simulink model "PV_Series_Parallel_Array"  (R2020a)
settings: Solver=VariableStepAuto  StartTime=0.0  StopTime=5  RelTol=1e-3
values from neighbouring files (symbols this model uses):
  Eg = 1.1    [data.m]
  Isc = 8.21    [data.m]
  k = 1.38*((10)^-23)    (= 1.38e-23)    [data.m]
  ki = 0.0032    [data.m]
  n = 1.3    [data.m]
  Ns = 54    [data.m]
  q = 1.6*((10)^-19)    (= 1.6e-19)    [data.m]
  Rs = 0.221    [data.m]
  Rsh = 415.405    [data.m]
  Tn = 298    [data.m]
  Voc = 32.9    [data.m]
libraries: powerlib x25
settings Model: Creator=Khojasteh Mirza  LastModifiedBy=Khojasteh Mirza

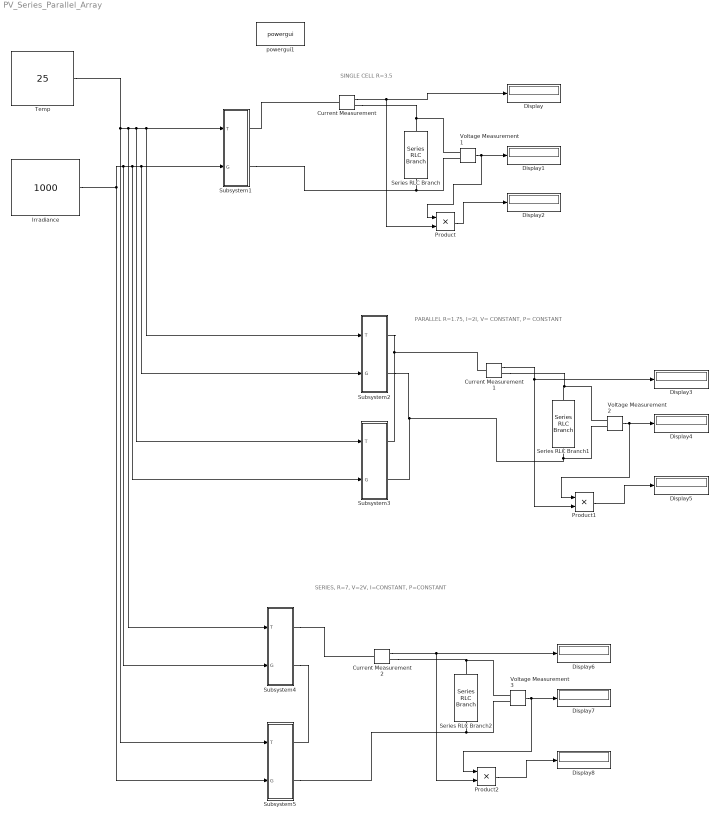
== system PV_Series_Parallel_Array ==
  note: SERIES, R=7, V=2V, I=CONSTANT, P=CONSTANT
  note: PARALLEL R=1.75, I=2I, V= CONSTANT, P= CONSTANT
  note: SINGLE CELL R=3.5
  Current Measurement : powerlib/Measurements/Current Measurement  PhasorSimulation=off  OutputType=Complex  PSBequivalent=0
  Current Measurement1 : powerlib/Measurements/Current Measurement  PhasorSimulation=off  OutputType=Complex  PSBequivalent=0
  Current Measurement2 : powerlib/Measurements/Current Measurement  PhasorSimulation=off  OutputType=Complex  PSBequivalent=0
  Display{,1..8} (9 alike) : Display
  Irradiance : Constant  Value=1000
  Product : Product
  Product1 : Product
  Product2 : Product
  Series RLC Branch : powerlib/Elements/Series RLC Branch  LConnTagsString=__new0  RConnTagsString=__new0  BranchType=R  Resistance=3.5  Inductance=1e-3  SetiL0=off  InitialCurrent=0  Capacitance=1e-6  Setx0=off  InitialVoltage=0  Measurements=None
  Series RLC Branch1 : powerlib/Elements/Series RLC Branch  LConnTagsString=__new0  RConnTagsString=__new0  BranchType=R  Resistance=1.75  Inductance=1e-3  SetiL0=off  InitialCurrent=0  Capacitance=1e-6  Setx0=off  InitialVoltage=0  Measurements=None
  Series RLC Branch2 : powerlib/Elements/Series RLC Branch  LConnTagsString=__new0  RConnTagsString=__new0  BranchType=R  Resistance=7  Inductance=1e-3  SetiL0=off  InitialCurrent=0  Capacitance=1e-6  Setx0=off  InitialVoltage=0  Measurements=None
  Subsystem1 : Subsystem
  Subsystem2 : Subsystem
  Subsystem3 : Subsystem
  Subsystem4 : Subsystem
  Subsystem5 : Subsystem
  Temp : Constant  Value=25
  Voltage Measurement1 : powerlib/Measurements/Voltage Measurement  PhasorSimulation=off  OutputType=Complex  PSBequivalent=0
  Voltage Measurement2 : powerlib/Measurements/Voltage Measurement  PhasorSimulation=off  OutputType=Complex  PSBequivalent=0
  Voltage Measurement3 : powerlib/Measurements/Voltage Measurement  PhasorSimulation=off  OutputType=Complex  PSBequivalent=0
  powergui1 : powerlib/powergui  Priority=1  SimulationMode=Continuous  SampleTime=50e-6  frequency=60  Iterations=50  frequencyindice=0  Pbase=100e6  ErrMax=1e-4  UnitsV=kV  UnitsW=MW  buscounter=0  FunctionMessages=off  echomessages=off  EnableUseOfTLC=off  CurrentSourceSwitches=off  DisableSnubberDevices=off  DisableRonSwitches=off  DisableVfSwitches=off  DisplayEquations=off  AutomaticDiscreteSolvers=off  SolverType=Tustin/Backward Euler (TBE)  Interpol=off  ExternalGateDelay=off  methode=off  Ts=100  x0status=blocks  SPID=on  SwTol=0  HookPort=off  NonlinearTolerance=1e-4  nMaxIteration=100  ContinueOnMaxIteration=off  RestoreLinks=warning  ResistiveCurrentMeasurement=off  Frange=[0:2:500]  Ylog=off  Xlog=on  ShowGrid=off  save=off  variable=ZData  structure=0  ZoomFFT=off  StartTime=0.0  cycles=1  DisplayStyle=1  fundamental=60  FreqAxis=off  MaxFrequency=1000  frequencyindicesteady=1  RmsSteady=1  display=off
  wires:
  Voltage Measurement1/1 -> Product/1, Display1/1
  Current Measurement/1 -> Product/2, Display/1
  Product/1 -> Display2/1
  Irradiance/1 -> Subsystem3/2(G), Subsystem2/2(G), Subsystem1/2(G), Subsystem4/2(G), Subsystem5/2(G)
  Temp/1 -> Subsystem5/1(T), Subsystem4/1(T), Subsystem3/1(T), Subsystem2/1(T), Subsystem1/1(T)
  Product1/1 -> Display5/1
  Current Measurement1/1 -> Display3/1, Product1/2
  Voltage Measurement2/1 -> Display4/1, Product1/1
  Voltage Measurement3/1 -> Product2/1, Display7/1
  Current Measurement2/1 -> Product2/2, Display6/1
  Product2/1 -> Display8/1
  connections:
  Subsystem1/RConn2 -- Voltage Measurement1/LConn2 -- Series RLC Branch/RConn1
  Voltage Measurement1/LConn1 -- Current Measurement/RConn1 -- Series RLC Branch/LConn1
  Current Measurement/LConn1 -- Subsystem1/RConn1
  Subsystem2/RConn1 -- Subsystem3/RConn1 -- Current Measurement1/LConn1
  Voltage Measurement2/LConn2 -- Subsystem3/RConn2 -- Subsystem2/RConn2 -- Series RLC Branch1/RConn1
  Current Measurement1/RConn1 -- Voltage Measurement2/LConn1 -- Series RLC Branch1/LConn1
  Voltage Measurement3/LConn1 -- Current Measurement2/RConn1 -- Series RLC Branch2/LConn1
  Voltage Measurement3/LConn2 -- Subsystem5/RConn2 -- Series RLC Branch2/RConn1
  Subsystem4/RConn1 -- Current Measurement2/LConn1
  Subsystem4/RConn2 -- Subsystem5/RConn1

== system PV_Series_Parallel_Array/Subsystem1 ==
  T : Inport
  G : Inport  Port=2
  Controlled Current Source : powerlib/Electrical Sources/Controlled Current Source  Initialize=on  Source_Type=AC  Amplitude=0  Phase=0  Frequency=0  Measurements=None
  Diode : powerlib/Power Electronics/Diode  Ron=0.001  Lon=0  Vf=0.8  IC=0  UseSnubber=0  Rs=500  Cs=250e-9  Measurements=off
  PV Module : Subsystem
  Voltage Measurement : powerlib/Measurements/Voltage Measurement  PhasorSimulation=off  OutputType=Complex  PSBequivalent=0
  + : PMIOPort  Side=Right
  - : PMIOPort  Port=2  Side=Right
  wires:
  G/1 -> PV Module/2(G)
  Voltage Measurement/1 -> PV Module/3(Varray)
  T/1 -> PV Module/1(T)
  PV Module/1(I) -> Controlled Current Source/1
  connections:
  Voltage Measurement/LConn2 -- Diode/LConn1 -- Controlled Current Source/LConn1 -- -/RConn1
  Voltage Measurement/LConn1 -- Diode/RConn1 -- Controlled Current Source/RConn1 -- +/RConn1

== system PV_Series_Parallel_Array/Subsystem2 ==
  T : Inport
  G : Inport  Port=2
  Controlled Current Source : powerlib/Electrical Sources/Controlled Current Source  Initialize=on  Source_Type=AC  Amplitude=0  Phase=0  Frequency=0  Measurements=None
  Diode : powerlib/Power Electronics/Diode  Ron=0.001  Lon=0  Vf=0.8  IC=0  UseSnubber=0  Rs=500  Cs=250e-9  Measurements=off
  PV Module : Subsystem
  Voltage Measurement : powerlib/Measurements/Voltage Measurement  PhasorSimulation=off  OutputType=Complex  PSBequivalent=0
  + : PMIOPort  Side=Right
  - : PMIOPort  Port=2  Side=Right
  wires:
  PV Module/1(I) -> Controlled Current Source/1
  T/1 -> PV Module/1(T)
  Voltage Measurement/1 -> PV Module/3(Varray)
  G/1 -> PV Module/2(G)
  connections:
  Diode/RConn1 -- +/RConn1 -- Voltage Measurement/LConn1 -- Controlled Current Source/RConn1
  Diode/LConn1 -- Controlled Current Source/LConn1 -- -/RConn1 -- Voltage Measurement/LConn2

== system PV_Series_Parallel_Array/Subsystem3 ==
  T : Inport
  G : Inport  Port=2
  Controlled Current Source : powerlib/Electrical Sources/Controlled Current Source  Initialize=on  Source_Type=AC  Amplitude=0  Phase=0  Frequency=0  Measurements=None
  Diode : powerlib/Power Electronics/Diode  Ron=0.001  Lon=0  Vf=0.8  IC=0  UseSnubber=0  Rs=500  Cs=250e-9  Measurements=off
  PV Module : Subsystem
  Voltage Measurement : powerlib/Measurements/Voltage Measurement  PhasorSimulation=off  OutputType=Complex  PSBequivalent=0
  + : PMIOPort  Side=Right
  - : PMIOPort  Port=2  Side=Right
  wires:
  G/1 -> PV Module/2(G)
  Voltage Measurement/1 -> PV Module/3(Varray)
  T/1 -> PV Module/1(T)
  PV Module/1(I) -> Controlled Current Source/1
  connections:
  Voltage Measurement/LConn2 -- -/RConn1 -- Controlled Current Source/LConn1 -- Diode/LConn1
  Controlled Current Source/RConn1 -- Voltage Measurement/LConn1 -- +/RConn1 -- Diode/RConn1

== system PV_Series_Parallel_Array/Subsystem4 ==
  T : Inport
  G : Inport  Port=2
  Controlled Current Source : powerlib/Electrical Sources/Controlled Current Source  Initialize=on  Source_Type=AC  Amplitude=0  Phase=0  Frequency=0  Measurements=None
  Diode : powerlib/Power Electronics/Diode  Ron=0.001  Lon=0  Vf=0.8  IC=0  UseSnubber=0  Rs=500  Cs=250e-9  Measurements=off
  PV Module : Subsystem
  Voltage Measurement : powerlib/Measurements/Voltage Measurement  PhasorSimulation=off  OutputType=Complex  PSBequivalent=0
  + : PMIOPort  Side=Right
  - : PMIOPort  Port=2  Side=Right
  wires:
  G/1 -> PV Module/2(G)
  Voltage Measurement/1 -> PV Module/3(Varray)
  T/1 -> PV Module/1(T)
  PV Module/1(I) -> Controlled Current Source/1
  connections:
  Voltage Measurement/LConn2 -- -/RConn1 -- Controlled Current Source/LConn1 -- Diode/LConn1
  Controlled Current Source/RConn1 -- Voltage Measurement/LConn1 -- +/RConn1 -- Diode/RConn1

== system PV_Series_Parallel_Array/Subsystem5 ==
  T : Inport
  G : Inport  Port=2
  Controlled Current Source : powerlib/Electrical Sources/Controlled Current Source  Initialize=on  Source_Type=AC  Amplitude=0  Phase=0  Frequency=0  Measurements=None
  Diode : powerlib/Power Electronics/Diode  Ron=0.001  Lon=0  Vf=0.8  IC=0  UseSnubber=0  Rs=500  Cs=250e-9  Measurements=off
  PV Module : Subsystem
  Voltage Measurement : powerlib/Measurements/Voltage Measurement  PhasorSimulation=off  OutputType=Complex  PSBequivalent=0
  + : PMIOPort  Side=Right
  - : PMIOPort  Port=2  Side=Right
  wires:
  PV Module/1(I) -> Controlled Current Source/1
  T/1 -> PV Module/1(T)
  Voltage Measurement/1 -> PV Module/3(Varray)
  G/1 -> PV Module/2(G)
  connections:
  Diode/RConn1 -- +/RConn1 -- Voltage Measurement/LConn1 -- Controlled Current Source/RConn1
  Diode/LConn1 -- Controlled Current Source/LConn1 -- -/RConn1 -- Voltage Measurement/LConn2

== system PV_Series_Parallel_Array/Subsystem1/PV Module ==
  T : Inport
  G : Inport  Port=2
  Varray : Inport  Port=3
  Add : Sum
  Constant : Constant  Value=273
  PV Current : Subsystem
  Photo current : Subsystem
  Reverse Saturation Current : Subsystem
  Saturation Current : Subsystem
  Shunt Current : Subsystem
  I : Outport
  wires:
  Shunt Current/1(Ish) -> PV Current/4(Ish)
  Varray/1 -> Shunt Current/2(V), PV Current/1(V)
  Reverse Saturation Current/1(Irs) -> Saturation Current/2(Irs)
  Saturation Current/1(I_0) -> PV Current/3(I0)
  Constant/1 -> Add/2
  G/1 -> Photo current/2(G)
  T/1 -> Add/1
  PV Current/1(I) -> I/1, Shunt Current/1(I)
  Photo current/1(Iph) -> PV Current/5(Iph)
  Add/1 -> Saturation Current/1(T), Reverse Saturation Current/1(T), Photo current/1(T), PV Current/2(T)

== system PV_Series_Parallel_Array/Subsystem2/PV Module ==
  T : Inport
  G : Inport  Port=2
  Varray : Inport  Port=3
  Add : Sum
  Constant : Constant  Value=273
  PV Current : Subsystem
  Photo current : Subsystem
  Reverse Saturation Current : Subsystem
  Saturation Current : Subsystem
  Shunt Current : Subsystem
  I : Outport
  wires:
  Add/1 -> PV Current/2(T), Photo current/1(T), Reverse Saturation Current/1(T), Saturation Current/1(T)
  Photo current/1(Iph) -> PV Current/5(Iph)
  PV Current/1(I) -> Shunt Current/1(I), I/1
  T/1 -> Add/1
  G/1 -> Photo current/2(G)
  Constant/1 -> Add/2
  Saturation Current/1(I_0) -> PV Current/3(I0)
  Reverse Saturation Current/1(Irs) -> Saturation Current/2(Irs)
  Varray/1 -> PV Current/1(V), Shunt Current/2(V)
  Shunt Current/1(Ish) -> PV Current/4(Ish)

== system PV_Series_Parallel_Array/Subsystem3/PV Module ==
  T : Inport
  G : Inport  Port=2
  Varray : Inport  Port=3
  Add : Sum
  Constant : Constant  Value=273
  PV Current : Subsystem
  Photo current : Subsystem
  Reverse Saturation Current : Subsystem
  Saturation Current : Subsystem
  Shunt Current : Subsystem
  I : Outport
  wires:
  Shunt Current/1(Ish) -> PV Current/4(Ish)
  Varray/1 -> Shunt Current/2(V), PV Current/1(V)
  Reverse Saturation Current/1(Irs) -> Saturation Current/2(Irs)
  Saturation Current/1(I_0) -> PV Current/3(I0)
  Constant/1 -> Add/2
  G/1 -> Photo current/2(G)
  T/1 -> Add/1
  PV Current/1(I) -> I/1, Shunt Current/1(I)
  Photo current/1(Iph) -> PV Current/5(Iph)
  Add/1 -> Saturation Current/1(T), Reverse Saturation Current/1(T), Photo current/1(T), PV Current/2(T)

== system PV_Series_Parallel_Array/Subsystem4/PV Module ==
  T : Inport
  G : Inport  Port=2
  Varray : Inport  Port=3
  Add : Sum
  Constant : Constant  Value=273
  PV Current : Subsystem
  Photo current : Subsystem
  Reverse Saturation Current : Subsystem
  Saturation Current : Subsystem
  Shunt Current : Subsystem
  I : Outport
  wires:
  Shunt Current/1(Ish) -> PV Current/4(Ish)
  Varray/1 -> Shunt Current/2(V), PV Current/1(V)
  Reverse Saturation Current/1(Irs) -> Saturation Current/2(Irs)
  Saturation Current/1(I_0) -> PV Current/3(I0)
  Constant/1 -> Add/2
  G/1 -> Photo current/2(G)
  T/1 -> Add/1
  PV Current/1(I) -> I/1, Shunt Current/1(I)
  Photo current/1(Iph) -> PV Current/5(Iph)
  Add/1 -> Saturation Current/1(T), Reverse Saturation Current/1(T), Photo current/1(T), PV Current/2(T)

== system PV_Series_Parallel_Array/Subsystem5/PV Module ==
  T : Inport
  G : Inport  Port=2
  Varray : Inport  Port=3
  Add : Sum
  Constant : Constant  Value=273
  PV Current : Subsystem
  Photo current : Subsystem
  Reverse Saturation Current : Subsystem
  Saturation Current : Subsystem
  Shunt Current : Subsystem
  I : Outport
  wires:
  Add/1 -> PV Current/2(T), Photo current/1(T), Reverse Saturation Current/1(T), Saturation Current/1(T)
  Photo current/1(Iph) -> PV Current/5(Iph)
  PV Current/1(I) -> Shunt Current/1(I), I/1
  T/1 -> Add/1
  G/1 -> Photo current/2(G)
  Constant/1 -> Add/2
  Saturation Current/1(I_0) -> PV Current/3(I0)
  Reverse Saturation Current/1(Irs) -> Saturation Current/2(Irs)
  Varray/1 -> PV Current/1(V), Shunt Current/2(V)
  Shunt Current/1(Ish) -> PV Current/4(Ish)

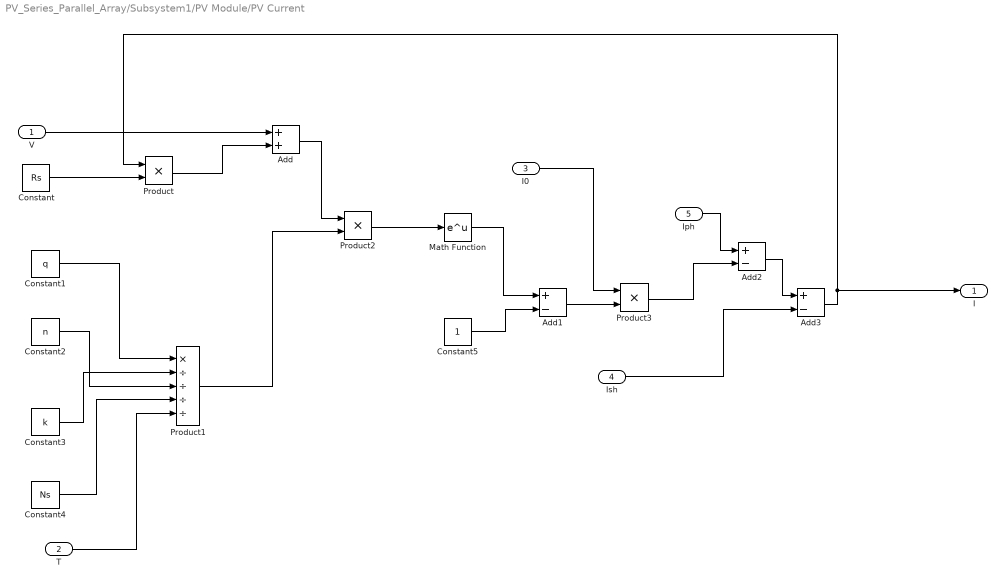
== system PV_Series_Parallel_Array/Subsystem1/PV Module/PV Current ==
  V : Inport
  T : Inport  Port=2
  I0 : Inport  Port=3
  Ish : Inport  Port=4
  Iph : Inport  Port=5
  Add : Sum
  Add1 : Sum  Inputs=+-
  Add2 : Sum  Inputs=+-
  Add3 : Sum  Inputs=+-
  Constant : Constant  Value=Rs
  Constant1 : Constant  Value=q
  Constant2 : Constant  Value=n
  Constant3 : Constant  Value=k
  Constant4 : Constant  Value=Ns
  Constant5 : Constant
  Math Function : Math  SaturateOnIntegerOverflow=on
  Product : Product
  Product1 : Product  Inputs=*////
  Product2 : Product
  Product3 : Product
  I : Outport
  wires:
  Constant3/1 -> Product1/2
  Constant/1 -> Product/2
  Math Function/1 -> Add1/1
  Iph/1 -> Add2/1
  Product2/1 -> Math Function/1
  I0/1 -> Product3/1
  Ish/1 -> Add3/2
  Product/1 -> Add/2
  Constant4/1 -> Product1/4
  Add/1 -> Product2/1
  Add3/1 -> I/1, Product/1
  Add1/1 -> Product3/2
  Constant2/1 -> Product1/3
  Add2/1 -> Add3/1
  T/1 -> Product1/5
  Product3/1 -> Add2/2
  V/1 -> Add/1
  Constant1/1 -> Product1/1
  Constant5/1 -> Add1/2
  Product1/1 -> Product2/2

== system PV_Series_Parallel_Array/Subsystem1/PV Module/Photo current ==
  T : Inport
  G : Inport  Port=2
  Add : Sum  Inputs=+-
  Add1 : Sum
  Constant : Constant  Value=298
  Constant1 : Constant  Value=ki
  Constant2 : Constant  Value=Isc
  Constant3 : Constant  Value=1000
  Product : Product
  Product1 : Product
  Product2 : Product  Inputs=*/
  Iph : Outport
  wires:
  Add/1 -> Product/1
  T/1 -> Add/1
  Constant2/1 -> Add1/1
  Constant/1 -> Add/2
  Product/1 -> Add1/2
  Constant1/1 -> Product/2
  G/1 -> Product1/1
  Constant3/1 -> Product2/2
  Add1/1 -> Product1/2
  Product1/1 -> Product2/1
  Product2/1 -> Iph/1

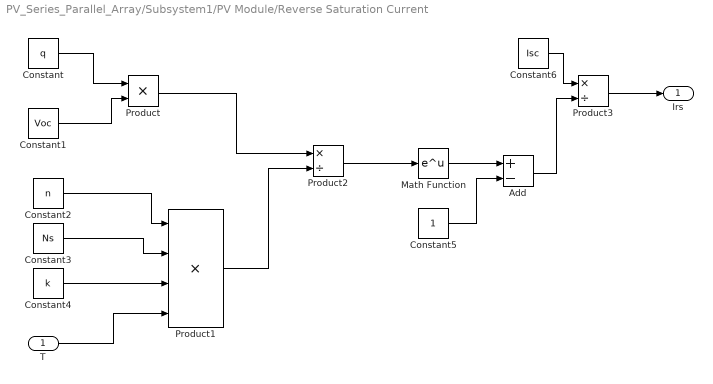
== system PV_Series_Parallel_Array/Subsystem1/PV Module/Reverse Saturation Current ==
  T : Inport
  Add : Sum  Inputs=+-
  Constant : Constant  Value=q
  Constant1 : Constant  Value=Voc
  Constant2 : Constant  Value=n
  Constant3 : Constant  Value=Ns
  Constant4 : Constant  Value=k
  Constant5 : Constant
  Constant6 : Constant  Value=Isc
  Math Function : Math  SaturateOnIntegerOverflow=on
  Product : Product
  Product1 : Product  Inputs=4
  Product2 : Product  Inputs=*/
  Product3 : Product  Inputs=*/
  Irs : Outport
  wires:
  Constant6/1 -> Product3/1
  Add/1 -> Product3/2
  Constant5/1 -> Add/2
  Constant3/1 -> Product1/2
  Product3/1 -> Irs/1
  Product1/1 -> Product2/2
  Math Function/1 -> Add/1
  Product/1 -> Product2/1
  Constant2/1 -> Product1/1
  Product2/1 -> Math Function/1
  Constant/1 -> Product/1
  Constant1/1 -> Product/2
  T/1 -> Product1/4
  Constant4/1 -> Product1/3

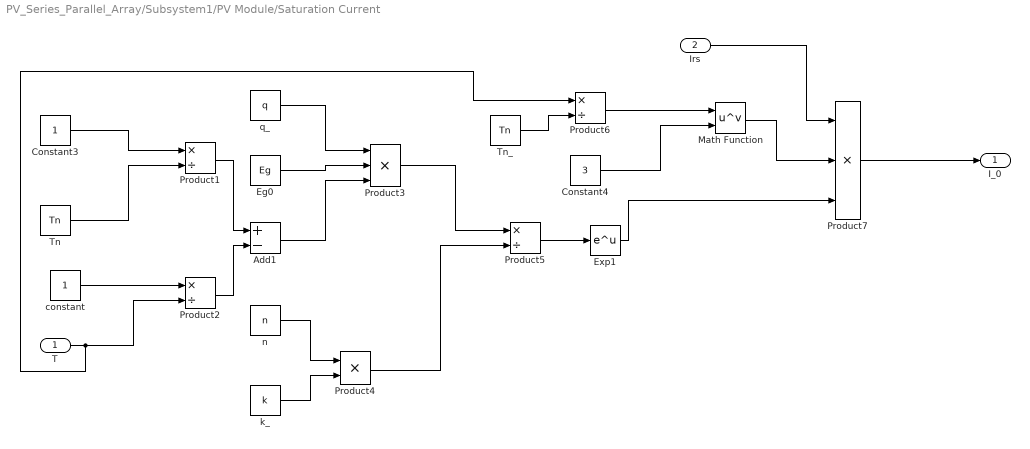
== system PV_Series_Parallel_Array/Subsystem1/PV Module/Saturation Current ==
  T : Inport
  Irs : Inport  Port=2
  Add1 : Sum  Inputs=+-
  Constant3 : Constant
  Constant4 : Constant  Value=3
  Eg0 : Constant  Value=Eg
  Exp1 : Math  SaturateOnIntegerOverflow=on
  Math Function : Math  Operator=pow  SaturateOnIntegerOverflow=on
  Product{1..2,5..6} (4 alike) : Product  Inputs=*/
  Product3 : Product  Inputs=***
  Product4 : Product  Inputs=**
  Product7 : Product  Inputs=3
  Tn : Constant  Value=Tn
  Tn_ : Constant  Value=Tn
  constant : Constant
  k_ : Constant  Value=k
  n : Constant  Value=n
  q_ : Constant  Value=q
  I_0 : Outport
  wires:
  T/1 -> Product2/2, Product6/1
  Product1/1 -> Add1/1
  constant/1 -> Product2/1
  Irs/1 -> Product7/1
  Tn_/1 -> Product6/2
  Product5/1 -> Exp1/1
  Product3/1 -> Product5/1
  q_/1 -> Product3/1
  Exp1/1 -> Product7/3
  Product2/1 -> Add1/2
  Product4/1 -> Product5/2
  Constant4/1 -> Math Function/2
  Math Function/1 -> Product7/2
  Tn/1 -> Product1/2
  Product6/1 -> Math Function/1
  k_/1 -> Product4/2
  Constant3/1 -> Product1/1
  Eg0/1 -> Product3/2
  n/1 -> Product4/1
  Add1/1 -> Product3/3
  Product7/1 -> I_0/1

== system PV_Series_Parallel_Array/Subsystem1/PV Module/Shunt Current ==
  I : Inport
  V : Inport  Port=2
  Add : Sum
  Constant : Constant  Value=Rs
  Constant1 : Constant  Value=Rsh
  Product : Product
  Product1 : Product  Inputs=*/
  Ish : Outport
  wires:
  Product1/1 -> Ish/1
  Constant/1 -> Product/2
  Constant1/1 -> Product1/2
  V/1 -> Add/2
  Product/1 -> Add/1
  Add/1 -> Product1/1
  I/1 -> Product/1

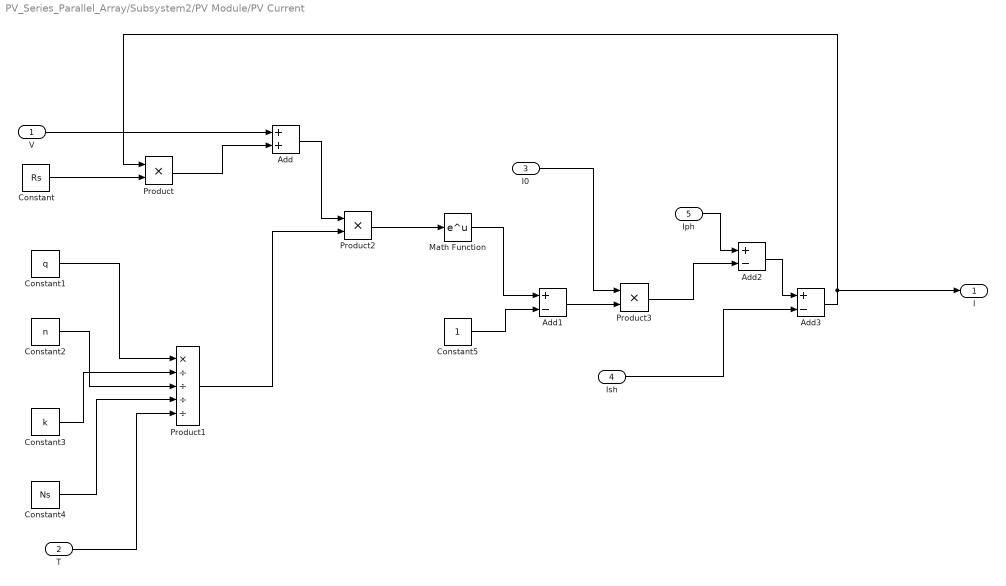
== system PV_Series_Parallel_Array/Subsystem2/PV Module/PV Current ==
  V : Inport
  T : Inport  Port=2
  I0 : Inport  Port=3
  Ish : Inport  Port=4
  Iph : Inport  Port=5
  Add : Sum
  Add1 : Sum  Inputs=+-
  Add2 : Sum  Inputs=+-
  Add3 : Sum  Inputs=+-
  Constant : Constant  Value=Rs
  Constant1 : Constant  Value=q
  Constant2 : Constant  Value=n
  Constant3 : Constant  Value=k
  Constant4 : Constant  Value=Ns
  Constant5 : Constant
  Math Function : Math  SaturateOnIntegerOverflow=on
  Product : Product
  Product1 : Product  Inputs=*////
  Product2 : Product
  Product3 : Product
  I : Outport
  wires:
  Product1/1 -> Product2/2
  Constant5/1 -> Add1/2
  Constant1/1 -> Product1/1
  V/1 -> Add/1
  Product3/1 -> Add2/2
  T/1 -> Product1/5
  Add2/1 -> Add3/1
  Constant2/1 -> Product1/3
  Add1/1 -> Product3/2
  Add3/1 -> Product/1, I/1
  Add/1 -> Product2/1
  Constant4/1 -> Product1/4
  Product/1 -> Add/2
  Ish/1 -> Add3/2
  I0/1 -> Product3/1
  Product2/1 -> Math Function/1
  Iph/1 -> Add2/1
  Math Function/1 -> Add1/1
  Constant/1 -> Product/2
  Constant3/1 -> Product1/2

== system PV_Series_Parallel_Array/Subsystem2/PV Module/Photo current ==
  T : Inport
  G : Inport  Port=2
  Add : Sum  Inputs=+-
  Add1 : Sum
  Constant : Constant  Value=298
  Constant1 : Constant  Value=ki
  Constant2 : Constant  Value=Isc
  Constant3 : Constant  Value=1000
  Product : Product
  Product1 : Product
  Product2 : Product  Inputs=*/
  Iph : Outport
  wires:
  Product2/1 -> Iph/1
  Product1/1 -> Product2/1
  Add1/1 -> Product1/2
  Constant3/1 -> Product2/2
  G/1 -> Product1/1
  Constant1/1 -> Product/2
  Product/1 -> Add1/2
  Constant/1 -> Add/2
  Constant2/1 -> Add1/1
  T/1 -> Add/1
  Add/1 -> Product/1

== system PV_Series_Parallel_Array/Subsystem2/PV Module/Reverse Saturation Current ==
  T : Inport
  Add : Sum  Inputs=+-
  Constant : Constant  Value=q
  Constant1 : Constant  Value=Voc
  Constant2 : Constant  Value=n
  Constant3 : Constant  Value=Ns
  Constant4 : Constant  Value=k
  Constant5 : Constant
  Constant6 : Constant  Value=Isc
  Math Function : Math  SaturateOnIntegerOverflow=on
  Product : Product
  Product1 : Product  Inputs=4
  Product2 : Product  Inputs=*/
  Product3 : Product  Inputs=*/
  Irs : Outport
  wires:
  Constant4/1 -> Product1/3
  T/1 -> Product1/4
  Constant1/1 -> Product/2
  Constant/1 -> Product/1
  Product2/1 -> Math Function/1
  Constant2/1 -> Product1/1
  Product/1 -> Product2/1
  Math Function/1 -> Add/1
  Product1/1 -> Product2/2
  Product3/1 -> Irs/1
  Constant3/1 -> Product1/2
  Constant5/1 -> Add/2
  Add/1 -> Product3/2
  Constant6/1 -> Product3/1

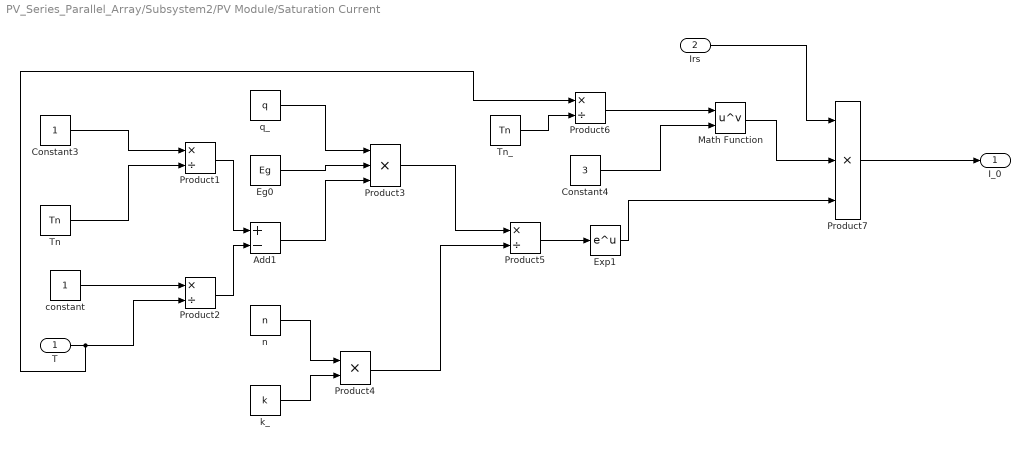
== system PV_Series_Parallel_Array/Subsystem2/PV Module/Saturation Current ==
  T : Inport
  Irs : Inport  Port=2
  Add1 : Sum  Inputs=+-
  Constant3 : Constant
  Constant4 : Constant  Value=3
  Eg0 : Constant  Value=Eg
  Exp1 : Math  SaturateOnIntegerOverflow=on
  Math Function : Math  Operator=pow  SaturateOnIntegerOverflow=on
  Product{1..2,5..6} (4 alike) : Product  Inputs=*/
  Product3 : Product  Inputs=***
  Product4 : Product  Inputs=**
  Product7 : Product  Inputs=3
  Tn : Constant  Value=Tn
  Tn_ : Constant  Value=Tn
  constant : Constant
  k_ : Constant  Value=k
  n : Constant  Value=n
  q_ : Constant  Value=q
  I_0 : Outport
  wires:
  Product7/1 -> I_0/1
  Add1/1 -> Product3/3
  n/1 -> Product4/1
  Eg0/1 -> Product3/2
  Constant3/1 -> Product1/1
  k_/1 -> Product4/2
  Product6/1 -> Math Function/1
  Tn/1 -> Product1/2
  Math Function/1 -> Product7/2
  Constant4/1 -> Math Function/2
  Product4/1 -> Product5/2
  Product2/1 -> Add1/2
  Exp1/1 -> Product7/3
  q_/1 -> Product3/1
  Product3/1 -> Product5/1
  Product5/1 -> Exp1/1
  Tn_/1 -> Product6/2
  Irs/1 -> Product7/1
  constant/1 -> Product2/1
  Product1/1 -> Add1/1
  T/1 -> Product6/1, Product2/2

== system PV_Series_Parallel_Array/Subsystem2/PV Module/Shunt Current ==
  I : Inport
  V : Inport  Port=2
  Add : Sum
  Constant : Constant  Value=Rs
  Constant1 : Constant  Value=Rsh
  Product : Product
  Product1 : Product  Inputs=*/
  Ish : Outport
  wires:
  I/1 -> Product/1
  Add/1 -> Product1/1
  Product/1 -> Add/1
  V/1 -> Add/2
  Constant1/1 -> Product1/2
  Constant/1 -> Product/2
  Product1/1 -> Ish/1

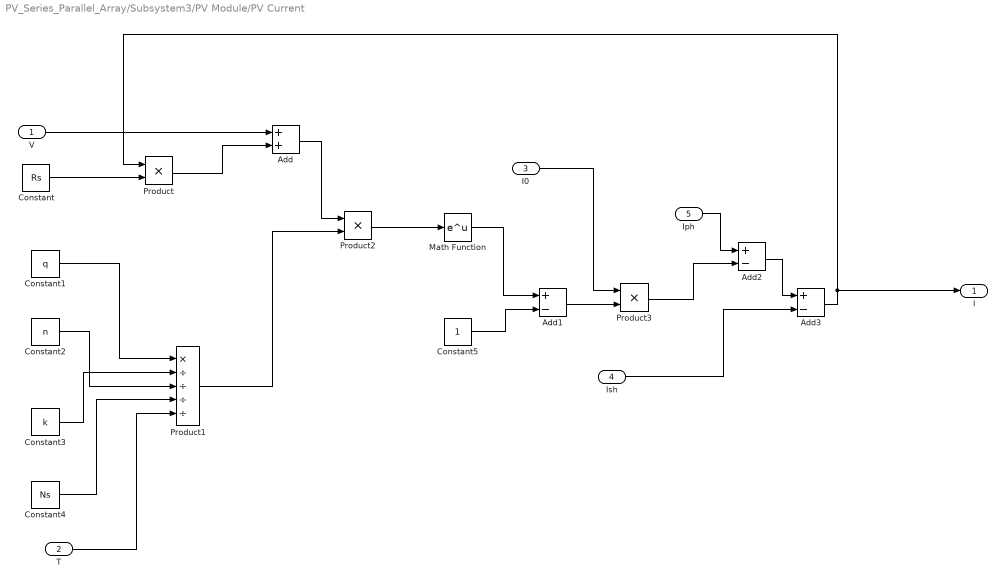
== system PV_Series_Parallel_Array/Subsystem3/PV Module/PV Current ==
  V : Inport
  T : Inport  Port=2
  I0 : Inport  Port=3
  Ish : Inport  Port=4
  Iph : Inport  Port=5
  Add : Sum
  Add1 : Sum  Inputs=+-
  Add2 : Sum  Inputs=+-
  Add3 : Sum  Inputs=+-
  Constant : Constant  Value=Rs
  Constant1 : Constant  Value=q
  Constant2 : Constant  Value=n
  Constant3 : Constant  Value=k
  Constant4 : Constant  Value=Ns
  Constant5 : Constant
  Math Function : Math  SaturateOnIntegerOverflow=on
  Product : Product
  Product1 : Product  Inputs=*////
  Product2 : Product
  Product3 : Product
  I : Outport
  wires:
  Constant3/1 -> Product1/2
  Constant/1 -> Product/2
  Math Function/1 -> Add1/1
  Iph/1 -> Add2/1
  Product2/1 -> Math Function/1
  I0/1 -> Product3/1
  Ish/1 -> Add3/2
  Product/1 -> Add/2
  Constant4/1 -> Product1/4
  Add/1 -> Product2/1
  Add3/1 -> I/1, Product/1
  Add1/1 -> Product3/2
  Constant2/1 -> Product1/3
  Add2/1 -> Add3/1
  T/1 -> Product1/5
  Product3/1 -> Add2/2
  V/1 -> Add/1
  Constant1/1 -> Product1/1
  Constant5/1 -> Add1/2
  Product1/1 -> Product2/2

== system PV_Series_Parallel_Array/Subsystem3/PV Module/Photo current ==
  T : Inport
  G : Inport  Port=2
  Add : Sum  Inputs=+-
  Add1 : Sum
  Constant : Constant  Value=298
  Constant1 : Constant  Value=ki
  Constant2 : Constant  Value=Isc
  Constant3 : Constant  Value=1000
  Product : Product
  Product1 : Product
  Product2 : Product  Inputs=*/
  Iph : Outport
  wires:
  Add/1 -> Product/1
  T/1 -> Add/1
  Constant2/1 -> Add1/1
  Constant/1 -> Add/2
  Product/1 -> Add1/2
  Constant1/1 -> Product/2
  G/1 -> Product1/1
  Constant3/1 -> Product2/2
  Add1/1 -> Product1/2
  Product1/1 -> Product2/1
  Product2/1 -> Iph/1

== system PV_Series_Parallel_Array/Subsystem3/PV Module/Reverse Saturation Current ==
  T : Inport
  Add : Sum  Inputs=+-
  Constant : Constant  Value=q
  Constant1 : Constant  Value=Voc
  Constant2 : Constant  Value=n
  Constant3 : Constant  Value=Ns
  Constant4 : Constant  Value=k
  Constant5 : Constant
  Constant6 : Constant  Value=Isc
  Math Function : Math  SaturateOnIntegerOverflow=on
  Product : Product
  Product1 : Product  Inputs=4
  Product2 : Product  Inputs=*/
  Product3 : Product  Inputs=*/
  Irs : Outport
  wires:
  Constant6/1 -> Product3/1
  Add/1 -> Product3/2
  Constant5/1 -> Add/2
  Constant3/1 -> Product1/2
  Product3/1 -> Irs/1
  Product1/1 -> Product2/2
  Math Function/1 -> Add/1
  Product/1 -> Product2/1
  Constant2/1 -> Product1/1
  Product2/1 -> Math Function/1
  Constant/1 -> Product/1
  Constant1/1 -> Product/2
  T/1 -> Product1/4
  Constant4/1 -> Product1/3

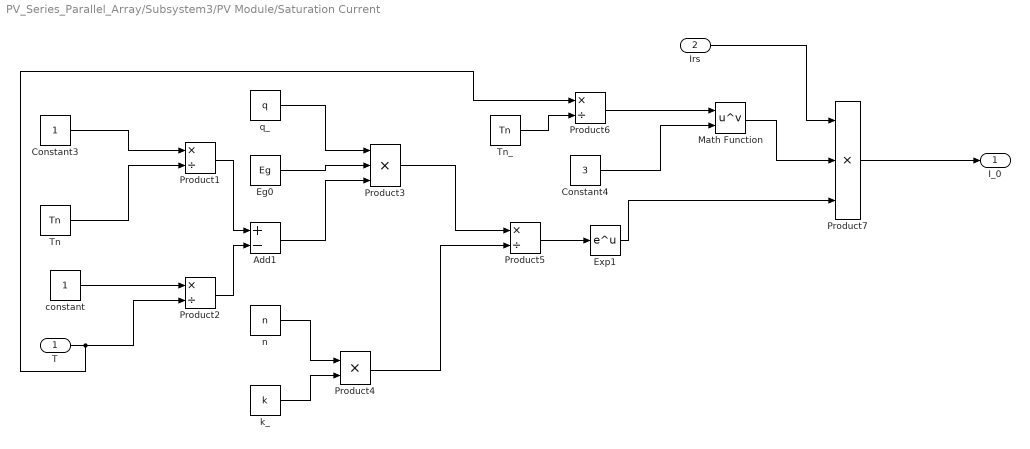
== system PV_Series_Parallel_Array/Subsystem3/PV Module/Saturation Current ==
  T : Inport
  Irs : Inport  Port=2
  Add1 : Sum  Inputs=+-
  Constant3 : Constant
  Constant4 : Constant  Value=3
  Eg0 : Constant  Value=Eg
  Exp1 : Math  SaturateOnIntegerOverflow=on
  Math Function : Math  Operator=pow  SaturateOnIntegerOverflow=on
  Product{1..2,5..6} (4 alike) : Product  Inputs=*/
  Product3 : Product  Inputs=***
  Product4 : Product  Inputs=**
  Product7 : Product  Inputs=3
  Tn : Constant  Value=Tn
  Tn_ : Constant  Value=Tn
  constant : Constant
  k_ : Constant  Value=k
  n : Constant  Value=n
  q_ : Constant  Value=q
  I_0 : Outport
  wires:
  T/1 -> Product2/2, Product6/1
  Product1/1 -> Add1/1
  constant/1 -> Product2/1
  Irs/1 -> Product7/1
  Tn_/1 -> Product6/2
  Product5/1 -> Exp1/1
  Product3/1 -> Product5/1
  q_/1 -> Product3/1
  Exp1/1 -> Product7/3
  Product2/1 -> Add1/2
  Product4/1 -> Product5/2
  Constant4/1 -> Math Function/2
  Math Function/1 -> Product7/2
  Tn/1 -> Product1/2
  Product6/1 -> Math Function/1
  k_/1 -> Product4/2
  Constant3/1 -> Product1/1
  Eg0/1 -> Product3/2
  n/1 -> Product4/1
  Add1/1 -> Product3/3
  Product7/1 -> I_0/1

== system PV_Series_Parallel_Array/Subsystem3/PV Module/Shunt Current ==
  I : Inport
  V : Inport  Port=2
  Add : Sum
  Constant : Constant  Value=Rs
  Constant1 : Constant  Value=Rsh
  Product : Product
  Product1 : Product  Inputs=*/
  Ish : Outport
  wires:
  Product1/1 -> Ish/1
  Constant/1 -> Product/2
  Constant1/1 -> Product1/2
  V/1 -> Add/2
  Product/1 -> Add/1
  Add/1 -> Product1/1
  I/1 -> Product/1

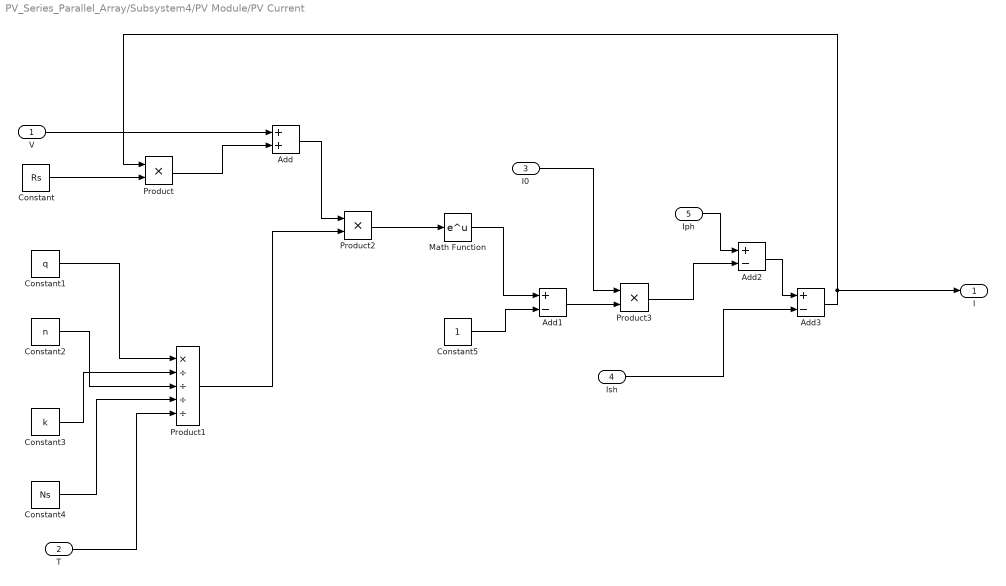
== system PV_Series_Parallel_Array/Subsystem4/PV Module/PV Current ==
  V : Inport
  T : Inport  Port=2
  I0 : Inport  Port=3
  Ish : Inport  Port=4
  Iph : Inport  Port=5
  Add : Sum
  Add1 : Sum  Inputs=+-
  Add2 : Sum  Inputs=+-
  Add3 : Sum  Inputs=+-
  Constant : Constant  Value=Rs
  Constant1 : Constant  Value=q
  Constant2 : Constant  Value=n
  Constant3 : Constant  Value=k
  Constant4 : Constant  Value=Ns
  Constant5 : Constant
  Math Function : Math  SaturateOnIntegerOverflow=on
  Product : Product
  Product1 : Product  Inputs=*////
  Product2 : Product
  Product3 : Product
  I : Outport
  wires:
  Constant3/1 -> Product1/2
  Constant/1 -> Product/2
  Math Function/1 -> Add1/1
  Iph/1 -> Add2/1
  Product2/1 -> Math Function/1
  I0/1 -> Product3/1
  Ish/1 -> Add3/2
  Product/1 -> Add/2
  Constant4/1 -> Product1/4
  Add/1 -> Product2/1
  Add3/1 -> I/1, Product/1
  Add1/1 -> Product3/2
  Constant2/1 -> Product1/3
  Add2/1 -> Add3/1
  T/1 -> Product1/5
  Product3/1 -> Add2/2
  V/1 -> Add/1
  Constant1/1 -> Product1/1
  Constant5/1 -> Add1/2
  Product1/1 -> Product2/2

== system PV_Series_Parallel_Array/Subsystem4/PV Module/Photo current ==
  T : Inport
  G : Inport  Port=2
  Add : Sum  Inputs=+-
  Add1 : Sum
  Constant : Constant  Value=298
  Constant1 : Constant  Value=ki
  Constant2 : Constant  Value=Isc
  Constant3 : Constant  Value=1000
  Product : Product
  Product1 : Product
  Product2 : Product  Inputs=*/
  Iph : Outport
  wires:
  Add/1 -> Product/1
  T/1 -> Add/1
  Constant2/1 -> Add1/1
  Constant/1 -> Add/2
  Product/1 -> Add1/2
  Constant1/1 -> Product/2
  G/1 -> Product1/1
  Constant3/1 -> Product2/2
  Add1/1 -> Product1/2
  Product1/1 -> Product2/1
  Product2/1 -> Iph/1

== system PV_Series_Parallel_Array/Subsystem4/PV Module/Reverse Saturation Current ==
  T : Inport
  Add : Sum  Inputs=+-
  Constant : Constant  Value=q
  Constant1 : Constant  Value=Voc
  Constant2 : Constant  Value=n
  Constant3 : Constant  Value=Ns
  Constant4 : Constant  Value=k
  Constant5 : Constant
  Constant6 : Constant  Value=Isc
  Math Function : Math  SaturateOnIntegerOverflow=on
  Product : Product
  Product1 : Product  Inputs=4
  Product2 : Product  Inputs=*/
  Product3 : Product  Inputs=*/
  Irs : Outport
  wires:
  Constant6/1 -> Product3/1
  Add/1 -> Product3/2
  Constant5/1 -> Add/2
  Constant3/1 -> Product1/2
  Product3/1 -> Irs/1
  Product1/1 -> Product2/2
  Math Function/1 -> Add/1
  Product/1 -> Product2/1
  Constant2/1 -> Product1/1
  Product2/1 -> Math Function/1
  Constant/1 -> Product/1
  Constant1/1 -> Product/2
  T/1 -> Product1/4
  Constant4/1 -> Product1/3

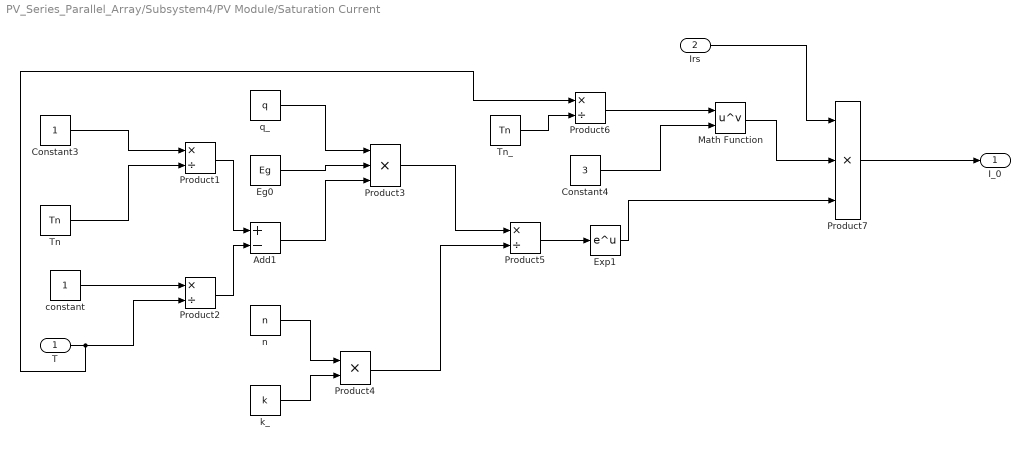
== system PV_Series_Parallel_Array/Subsystem4/PV Module/Saturation Current ==
  T : Inport
  Irs : Inport  Port=2
  Add1 : Sum  Inputs=+-
  Constant3 : Constant
  Constant4 : Constant  Value=3
  Eg0 : Constant  Value=Eg
  Exp1 : Math  SaturateOnIntegerOverflow=on
  Math Function : Math  Operator=pow  SaturateOnIntegerOverflow=on
  Product{1..2,5..6} (4 alike) : Product  Inputs=*/
  Product3 : Product  Inputs=***
  Product4 : Product  Inputs=**
  Product7 : Product  Inputs=3
  Tn : Constant  Value=Tn
  Tn_ : Constant  Value=Tn
  constant : Constant
  k_ : Constant  Value=k
  n : Constant  Value=n
  q_ : Constant  Value=q
  I_0 : Outport
  wires:
  T/1 -> Product2/2, Product6/1
  Product1/1 -> Add1/1
  constant/1 -> Product2/1
  Irs/1 -> Product7/1
  Tn_/1 -> Product6/2
  Product5/1 -> Exp1/1
  Product3/1 -> Product5/1
  q_/1 -> Product3/1
  Exp1/1 -> Product7/3
  Product2/1 -> Add1/2
  Product4/1 -> Product5/2
  Constant4/1 -> Math Function/2
  Math Function/1 -> Product7/2
  Tn/1 -> Product1/2
  Product6/1 -> Math Function/1
  k_/1 -> Product4/2
  Constant3/1 -> Product1/1
  Eg0/1 -> Product3/2
  n/1 -> Product4/1
  Add1/1 -> Product3/3
  Product7/1 -> I_0/1

== system PV_Series_Parallel_Array/Subsystem4/PV Module/Shunt Current ==
  I : Inport
  V : Inport  Port=2
  Add : Sum
  Constant : Constant  Value=Rs
  Constant1 : Constant  Value=Rsh
  Product : Product
  Product1 : Product  Inputs=*/
  Ish : Outport
  wires:
  Product1/1 -> Ish/1
  Constant/1 -> Product/2
  Constant1/1 -> Product1/2
  V/1 -> Add/2
  Product/1 -> Add/1
  Add/1 -> Product1/1
  I/1 -> Product/1

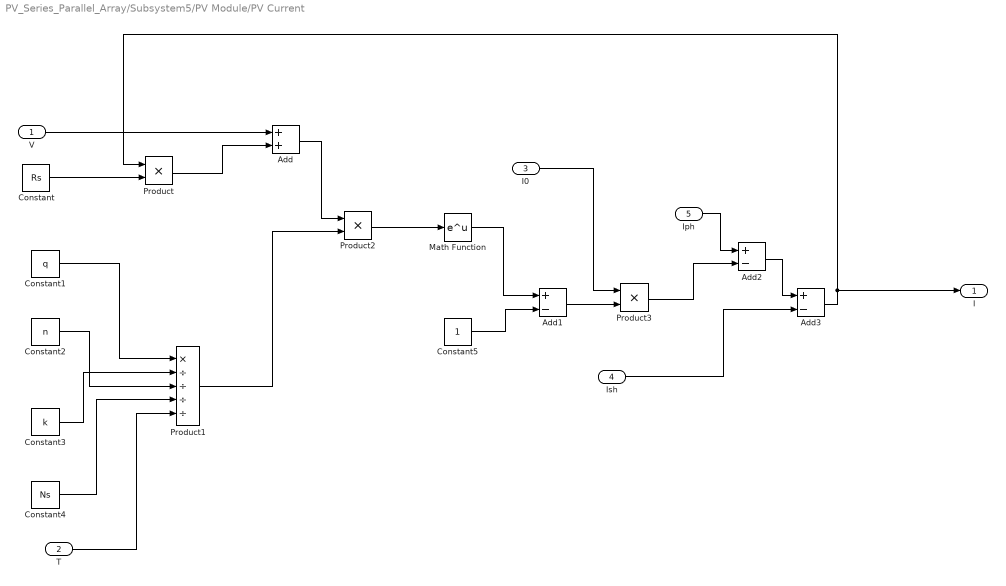
== system PV_Series_Parallel_Array/Subsystem5/PV Module/PV Current ==
  V : Inport
  T : Inport  Port=2
  I0 : Inport  Port=3
  Ish : Inport  Port=4
  Iph : Inport  Port=5
  Add : Sum
  Add1 : Sum  Inputs=+-
  Add2 : Sum  Inputs=+-
  Add3 : Sum  Inputs=+-
  Constant : Constant  Value=Rs
  Constant1 : Constant  Value=q
  Constant2 : Constant  Value=n
  Constant3 : Constant  Value=k
  Constant4 : Constant  Value=Ns
  Constant5 : Constant
  Math Function : Math  SaturateOnIntegerOverflow=on
  Product : Product
  Product1 : Product  Inputs=*////
  Product2 : Product
  Product3 : Product
  I : Outport
  wires:
  Product1/1 -> Product2/2
  Constant5/1 -> Add1/2
  Constant1/1 -> Product1/1
  V/1 -> Add/1
  Product3/1 -> Add2/2
  T/1 -> Product1/5
  Add2/1 -> Add3/1
  Constant2/1 -> Product1/3
  Add1/1 -> Product3/2
  Add3/1 -> Product/1, I/1
  Add/1 -> Product2/1
  Constant4/1 -> Product1/4
  Product/1 -> Add/2
  Ish/1 -> Add3/2
  I0/1 -> Product3/1
  Product2/1 -> Math Function/1
  Iph/1 -> Add2/1
  Math Function/1 -> Add1/1
  Constant/1 -> Product/2
  Constant3/1 -> Product1/2

== system PV_Series_Parallel_Array/Subsystem5/PV Module/Photo current ==
  T : Inport
  G : Inport  Port=2
  Add : Sum  Inputs=+-
  Add1 : Sum
  Constant : Constant  Value=298
  Constant1 : Constant  Value=ki
  Constant2 : Constant  Value=Isc
  Constant3 : Constant  Value=1000
  Product : Product
  Product1 : Product
  Product2 : Product  Inputs=*/
  Iph : Outport
  wires:
  Product2/1 -> Iph/1
  Product1/1 -> Product2/1
  Add1/1 -> Product1/2
  Constant3/1 -> Product2/2
  G/1 -> Product1/1
  Constant1/1 -> Product/2
  Product/1 -> Add1/2
  Constant/1 -> Add/2
  Constant2/1 -> Add1/1
  T/1 -> Add/1
  Add/1 -> Product/1

== system PV_Series_Parallel_Array/Subsystem5/PV Module/Reverse Saturation Current ==
  T : Inport
  Add : Sum  Inputs=+-
  Constant : Constant  Value=q
  Constant1 : Constant  Value=Voc
  Constant2 : Constant  Value=n
  Constant3 : Constant  Value=Ns
  Constant4 : Constant  Value=k
  Constant5 : Constant
  Constant6 : Constant  Value=Isc
  Math Function : Math  SaturateOnIntegerOverflow=on
  Product : Product
  Product1 : Product  Inputs=4
  Product2 : Product  Inputs=*/
  Product3 : Product  Inputs=*/
  Irs : Outport
  wires:
  Constant4/1 -> Product1/3
  T/1 -> Product1/4
  Constant1/1 -> Product/2
  Constant/1 -> Product/1
  Product2/1 -> Math Function/1
  Constant2/1 -> Product1/1
  Product/1 -> Product2/1
  Math Function/1 -> Add/1
  Product1/1 -> Product2/2
  Product3/1 -> Irs/1
  Constant3/1 -> Product1/2
  Constant5/1 -> Add/2
  Add/1 -> Product3/2
  Constant6/1 -> Product3/1

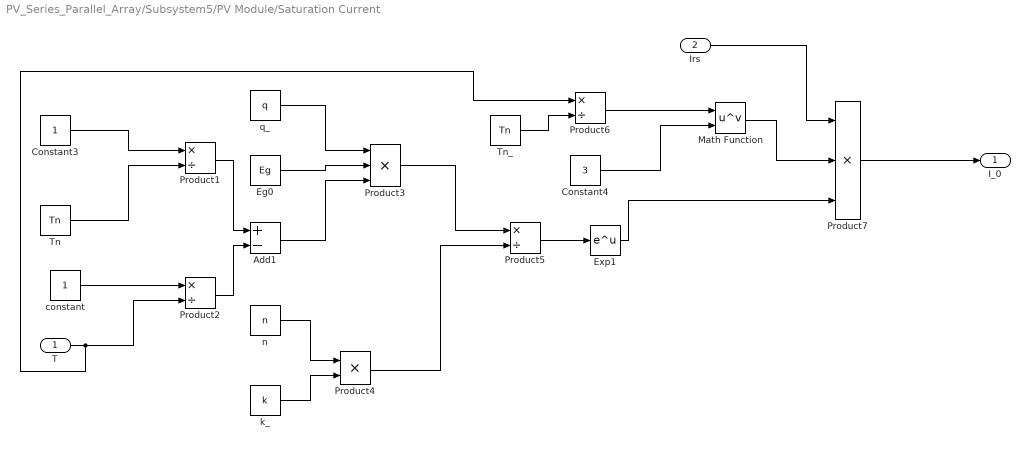
== system PV_Series_Parallel_Array/Subsystem5/PV Module/Saturation Current ==
  T : Inport
  Irs : Inport  Port=2
  Add1 : Sum  Inputs=+-
  Constant3 : Constant
  Constant4 : Constant  Value=3
  Eg0 : Constant  Value=Eg
  Exp1 : Math  SaturateOnIntegerOverflow=on
  Math Function : Math  Operator=pow  SaturateOnIntegerOverflow=on
  Product{1..2,5..6} (4 alike) : Product  Inputs=*/
  Product3 : Product  Inputs=***
  Product4 : Product  Inputs=**
  Product7 : Product  Inputs=3
  Tn : Constant  Value=Tn
  Tn_ : Constant  Value=Tn
  constant : Constant
  k_ : Constant  Value=k
  n : Constant  Value=n
  q_ : Constant  Value=q
  I_0 : Outport
  wires:
  Product7/1 -> I_0/1
  Add1/1 -> Product3/3
  n/1 -> Product4/1
  Eg0/1 -> Product3/2
  Constant3/1 -> Product1/1
  k_/1 -> Product4/2
  Product6/1 -> Math Function/1
  Tn/1 -> Product1/2
  Math Function/1 -> Product7/2
  Constant4/1 -> Math Function/2
  Product4/1 -> Product5/2
  Product2/1 -> Add1/2
  Exp1/1 -> Product7/3
  q_/1 -> Product3/1
  Product3/1 -> Product5/1
  Product5/1 -> Exp1/1
  Tn_/1 -> Product6/2
  Irs/1 -> Product7/1
  constant/1 -> Product2/1
  Product1/1 -> Add1/1
  T/1 -> Product6/1, Product2/2

== system PV_Series_Parallel_Array/Subsystem5/PV Module/Shunt Current ==
  I : Inport
  V : Inport  Port=2
  Add : Sum
  Constant : Constant  Value=Rs
  Constant1 : Constant  Value=Rsh
  Product : Product
  Product1 : Product  Inputs=*/
  Ish : Outport
  wires:
  I/1 -> Product/1
  Add/1 -> Product1/1
  Product/1 -> Add/1
  V/1 -> Add/2
  Constant1/1 -> Product1/2
  Constant/1 -> Product/2
  Product1/1 -> Ish/1
